simulink model "PI"  (Simulink 9.3)
settings: Solver=ode5  StartTime=0.0  StopTime=500  FixedStep=0.1  RelTol=1e-3  EnableMultiTasking=on
undefined symbols (not defined in the file): sigbuilder_block
libraries: fuzblock x1
settings Model: Creator=lemin  LastModifiedBy=forev
settings DataIOCC: LimitDataPoints=on
settings OptimizationCC: ExpressionDepthLimit=2147483647
settings DebuggingCC: SolverPrmCheckMsg=warning  StateNameClashWarn=warning  SFExecutionAtInitializationDiag=warning
settings GRTTargetCC: GeneratePreprocessorConditionals=Disable all

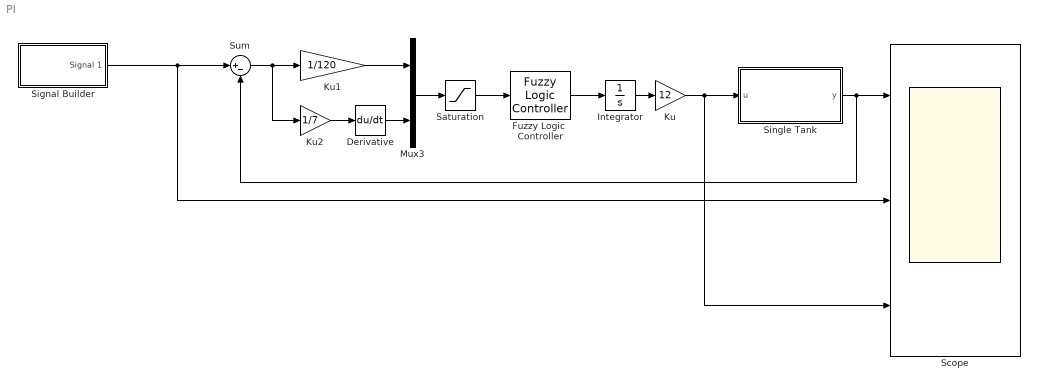
== system PI ==
  Derivative : Derivative
  Fuzzy Logic  Controller : fuzblock/Fuzzy Logic  Controller  FIS='PI.fis'  OutputSampleNumber=101  DataType=double  FuzzifiedInputs=off  RuleFiringStrengths=off  RuleOutputs=off  AggregatedOutputs=off  SimulateUsing=Interpreted execution  OutOfRangeInputValueMessage=warning  NoRuleFiredMessage=warning  EmptyOutputFuzzySetMessage=warning
  Integrator : Integrator  LimitOutput=on  UpperSaturationLimit=1  LowerSaturationLimit=0
  Ku : Gain  Gain=12
  Ku1 : Gain  Gain=1/120
  Ku2 : Gain  Gain=1/7
  Mux3 : Mux  Inputs=2
  Saturation : Saturate
  Scope : Scope  NumInputPorts=3
  Signal Builder : Subsystem  Tag=STV Subsys  LoadFcn=sigbuilder_block('load',[5.4 30 1141.2 522.6 ]);  StartFcn=sigbuilder_block('start');  StopFcn=sigbuilder_block('stop');  ClipboardFcn=sigbuilder_block('clipboard');  mask(Sigbuilder block){tuvar=[0:10]}
      mask help: Simulink:masks:SigbuilderBlock_MD
      mask init:
      | if ~strcmp(get_param(bdroot(gcbh),'SimulationStatus'),'stopped') tuvar = sigbuilder_block('maskInit'); end
      settings: CopyFcn=sigbuilder_block('copy');  DeleteFcn=sigbuilder_block('delete');  ModelCloseFcn=sigbuilder_block('modelClose');  PreSaveFcn=sigbuilder_block('preSave');  PauseFcn=sigbuilder_block('pause');  ContinueFcn=sigbuilder_block('continue');  NameChangeFcn=sigbuilder_block('namechange');  OpenFcn=sigbuilder_block('open',[5.4 30 1141.2 522.6 ]);  CloseFcn=sigbuilder_block('close');
      mask Display: plot(0, 0, 100, 100,[2, 2, 32, 32, 2], [68, 8, 8, 68, 68],[32, 2], [38, 38], [32, 19, 2],[53, 60, 44], [32, 17, 17, 2],[16, 16, 31, 31]);txt = getActiveGroup(gcbh);text(2, 100, txt,'verticalAlignment', 'top');
  Single Tank : Subsystem  mask{A=200, b=1.5, g=981, C=0.8, k=60, y0=0}
      mask prompts: A "Tiet dien ngang cua bon"; b "Tiet dien van xa"; g "gia toc trong truong"; C "He so xa"; k "He so cong suat bom"; y0 "vi tri nuoc ban dau"
  Sum : Sum  Inputs=|+-
  wires:
  Sum/1 -> Ku2/1, Ku1/1
  Ku2/1 -> Derivative/1
  Derivative/1 -> Mux3/2
  Ku1/1 -> Mux3/1
  Single Tank/1("y ") -> Scope/1, Sum/2
  Saturation/1 -> Fuzzy Logic  Controller/1
  Mux3/1 -> Saturation/1
  Signal Builder/1(Signal 1) -> Scope/2, Sum/1
  Integrator/1 -> Ku/1
  Ku/1 -> Scope/3, Single Tank/1("u ")
  Fuzzy Logic  Controller/1 -> Integrator/1

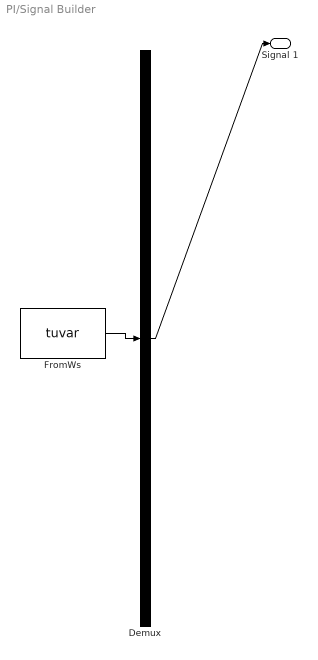
== system PI/Signal Builder ==
  Demux : Demux  Tag=STV Demux  Outputs=1
  FromWs : FromWorkspace  Tag=STV FromWs  VariableName=tuvar  SampleTime=0  SigBuilderData=DataTag0  VnvData=DataTag1
      SigBuilderData=|
      | common.afterFinalStr = 'Extrapolate'
      | common.sampleTime = 0
      | dataSet.timeRange = [0 500]
      | dataSet.name = 'Group 1'
      | sbobj.Groups.Name = 'Group 1'
      | sbobj.Groups.Signals.Name = 'Signal 1'
      | sbobj.Groups.Signals.XData = [0 3 3 32 62 62 99.5 132 132 148 269 269 331 397 397 464.5 500]
      | sbobj.Groups.Signals.YData = [1 1 111 111 111 39 39 39 61.5 61.5 61.5 110.5 110.5 110.5 33.5 33.5 33.5]
      | sbobj.Groups.TimeRange = [0 500]
  Signal 1 : Outport  Tag=STV Outport
  wires:
  FromWs/1 -> Demux/1
  Demux/1 -> Signal 1/1

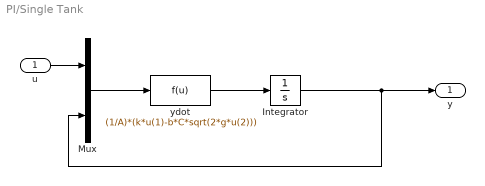
== system PI/Single Tank ==
  "u " : Inport
  Integrator : Integrator  InitialCondition=y0
  Mux : Mux  Inputs=2
  "ydot " : Fcn  Expr=(1/A)*(k*u(1)-b*C*sqrt(2*g*u(2)))
  "y " : Outport
  wires:
  "ydot "/1 -> Integrator/1
  Integrator/1 -> Mux/2, "y "/1
  "u "/1 -> Mux/1
  Mux/1 -> "ydot "/1
